simulink model "simulink_2a"  (R2018a)
settings: Solver=VariableStepAuto  StartTime=0.0  StopTime=1  RelTol=1e-3
values from neighbouring files (symbols this model uses):
  a1 = a(2)    [inicio_simulink.m]
  a2 = a(3)    [inicio_simulink.m]
  a3 = a(4)    [inicio_simulink.m]
  a4 = a(5)    [inicio_simulink.m]
  a5 = a(6)    [inicio_simulink.m]
  a6 = a(7)    [inicio_simulink.m]
  b0 = b(1)    [inicio_simulink.m]
  b1 = b(2)    [inicio_simulink.m]
  b2 = b(3)    [inicio_simulink.m]
  b3 = b(4)    [inicio_simulink.m]
  b4 = b(5)    [inicio_simulink.m]
  b5 = b(6)    [inicio_simulink.m]
  b6 = b(7)    [inicio_simulink.m]
settings Model: Creator=JORGE  LastModifiedBy=JORGE

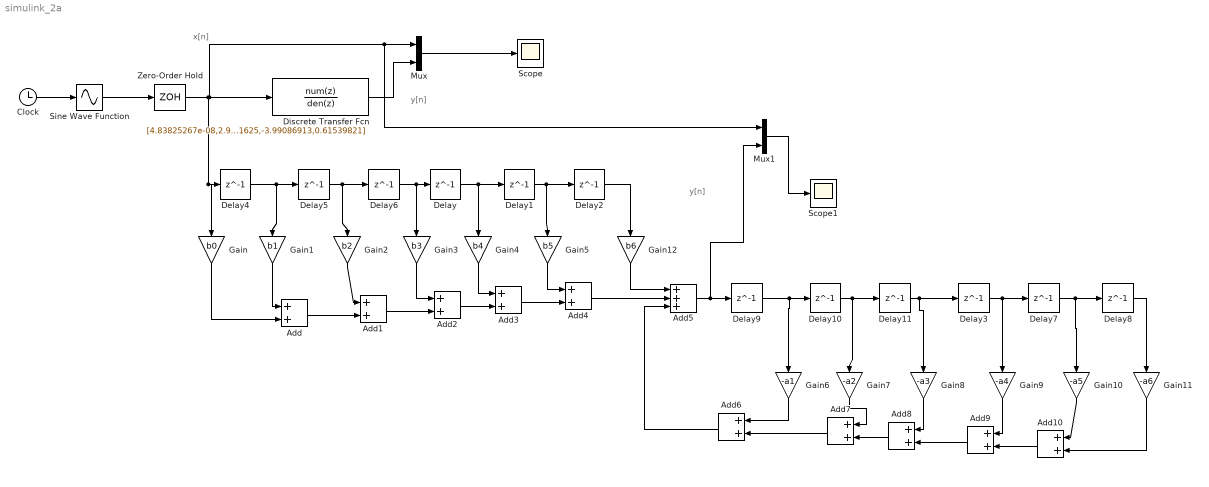
== system simulink_2a ==
  note: y[n]
  note: x[n]
  note: y[n]
  Add{,1..4,6..10} (10 alike) : Sum
  Add5 : Sum  Inputs=+++
  Clock : Clock
  Delay{,1..11} (12 alike) : Delay  DelayLength=1  SampleTime=1/500
  Discrete Transfer Fcn : DiscreteTransferFcn  Numerator=[4.83825267e-08,2.90295160e-07,7.25737900e-07,9.67650534e-07,7.257379e-07,2.90295160e-07,4.83825267e-08]  Denominator=[ 1,-5.51498094,12.69112968,-15.59729098,10.79661625,-3.99086913,0.61539821]
  Gain : Gain  Gain=b0
  Gain1 : Gain  Gain=b1
  Gain10 : Gain  Gain=-a5
  Gain11 : Gain  Gain=-a6
  Gain12 : Gain  Gain=b6
  Gain2 : Gain  Gain=b2
  Gain3 : Gain  Gain=b3
  Gain4 : Gain  Gain=b4
  Gain5 : Gain  Gain=b5
  Gain6 : Gain  Gain=-a1
  Gain7 : Gain  Gain=-a2
  Gain8 : Gain  Gain=-a3
  Gain9 : Gain  Gain=-a4
  Mux : Mux  Inputs=2
  Mux1 : Mux  Inputs=2
  Scope : Scope
  Scope1 : Scope
  Sine Wave Function : Sin  TimeSource=Use external signal  Frequency=5*(2*pi)  SampleTime=0
  Zero-Order Hold : ZeroOrderHold  SampleTime=1/500
  wires:
  Zero-Order Hold/1 -> Gain/1, Delay4/1, Mux1/1, Mux/1, Discrete Transfer Fcn/1
  Sine Wave Function/1 -> Zero-Order Hold/1
  Clock/1 -> Sine Wave Function/1
  Discrete Transfer Fcn/1 -> Mux/2
  Mux/1 -> Scope/1
  Delay1/1 -> Gain5/1, Delay2/1
  Delay4/1 -> Gain1/1, Delay5/1
  Delay5/1 -> Gain2/1, Delay6/1
  Delay6/1 -> Gain3/1, Delay/1
  Add/1 -> Add1/2
  Add1/1 -> Add2/2
  Add2/1 -> Add3/2
  Add3/1 -> Add4/2
  Add4/1 -> Add5/2
  Add5/1 -> Mux1/2, Delay9/1
  Add10/1 -> Add9/2
  Add9/1 -> Add8/2
  Add8/1 -> Add7/2
  Add7/1 -> Add6/2
  Add6/1 -> Add5/3
  Gain/1 -> Add/2
  Gain1/1 -> Add/1
  Gain2/1 -> Add1/1
  Gain3/1 -> Add2/1
  Gain4/1 -> Add3/1
  Delay/1 -> Delay1/1, Gain4/1
  Gain5/1 -> Add4/1
  Delay9/1 -> Gain6/1, Delay10/1
  Delay10/1 -> Gain7/1, Delay11/1
  Delay7/1 -> Gain10/1, Delay8/1
  Delay3/1 -> Gain9/1, Delay7/1
  Delay11/1 -> Gain8/1, Delay3/1
  Delay8/1 -> Gain11/1
  Gain11/1 -> Add10/2
  Gain10/1 -> Add10/1
  Gain9/1 -> Add9/1
  Gain8/1 -> Add8/1
  Gain7/1 -> Add7/1
  Gain6/1 -> Add6/1
  Delay2/1 -> Gain12/1
  Gain12/1 -> Add5/1
  Mux1/1 -> Scope1/1
